simulink model "power_measure"  (Simulink 8.1)
settings: Solver=ode45  StartTime=0.0  StopTime=0.5  RelTol=1e-3
values from neighbouring files (symbols this model uses):
  sample = 10e-5    (= 0.0001)    [Symmetry_ini_COPY.m]    (also in animated_norms.m)
libraries: commsequence2 x12, powerlib x8, dspxfrm3 x6, aerolibconvert2 x2
settings Model: Creator=Neukirchner László  LastModifiedBy=Neukirchner László
settings DataIOCC: SignalLoggingSaveFormat=Dataset
settings OptimizationCC: ExpressionDepthLimit=128
settings DebuggingCC: FcnCallInpInsideContextMsg=EnableAllAsError
settings GRTTargetCC: CombineOutputUpdateFcns=on  GRTInterface=off

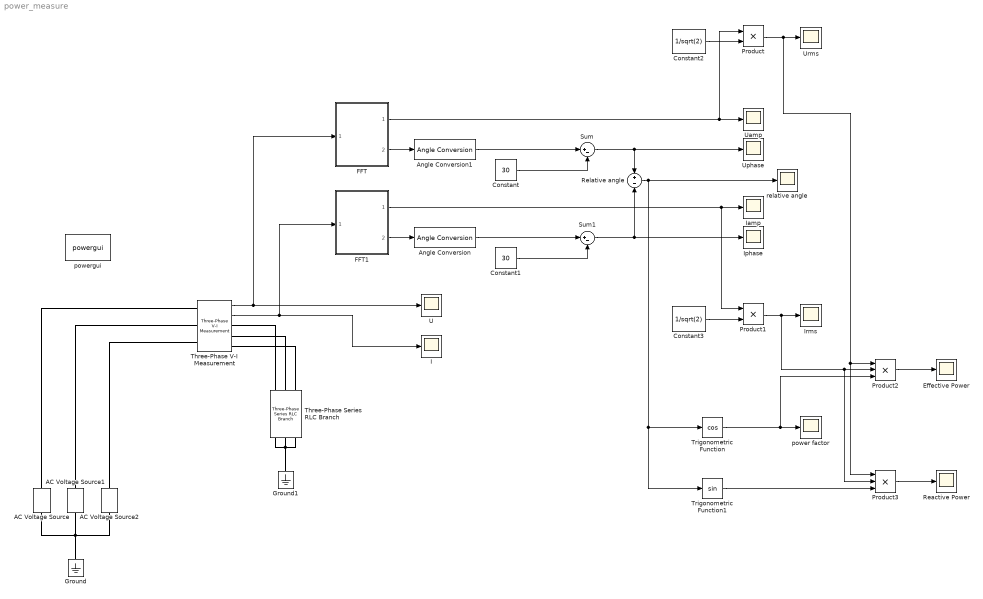
== system power_measure ==
  AC Voltage Source : powerlib/Electrical Sources/AC Voltage Source  Amplitude=325  Phase=0  Frequency=50  SampleTime=0  Measurements=None
  AC Voltage Source1 : powerlib/Electrical Sources/AC Voltage Source  Amplitude=325  Phase=-120  Frequency=50  SampleTime=0  Measurements=None
  AC Voltage Source2 : powerlib/Electrical Sources/AC Voltage Source  Amplitude=325  Phase=-240  Frequency=50  SampleTime=0  Measurements=None
  Angle Conversion : aerolibconvert2/Angle Conversion  IU=rad  OU=deg
  Angle Conversion1 : aerolibconvert2/Angle Conversion  IU=rad  OU=deg
  Constant : Constant  Value=30
  Constant1 : Constant  Value=30
  Constant2 : Constant  Value=1/sqrt(2)
  Constant3 : Constant  Value=1/sqrt(2)
  Effective Power : Scope
      settings: SaveName=ScopeData10
  FFT : Subsystem
  FFT1 : Subsystem
  Ground : powerlib/Elements/Ground  LConnTagsString=a
  Ground1 : powerlib/Elements/Ground  LConnTagsString=a
  I : Scope
  Iamp : Scope
      settings: SaveName=ScopeData4
  Iphase : Scope
      settings: SaveName=ScopeData5
  Irms : Scope
      settings: SaveName=ScopeData9
  Product : Product
  Product1 : Product
  Product2 : Product  Inputs=3
  Product3 : Product  Inputs=3
  Reactive Power : Scope
      settings: SaveName=ScopeData11
  Relative angle : Sum  Inputs=+|-
  Sum : Sum  Inputs=|+-
  Sum1 : Sum  Inputs=|+-
  Three-Phase Series RLC Branch : powerlib/Elements/Three-Phase Series RLC Branch  LConnTagsString=A|B|C  RConnTagsString=A|B|C  BranchType=RL  Resistance=100  Inductance=1e-1  Capacitance=1e-3  Measurements=None
  Three-Phase V-I Measurement : powerlib/Measurements/Three-Phase V-I Measurement  VoltageMeasurement=phase-to-ground  SetLabelV=off  LabelV=Vabc  Vpu=off  VpuLL=off  CurrentMeasurement=yes  SetLabelI=off  LabelI=Iabc  Ipu=off  Pbase=100e6  Vbase=500e3  OutputType=Complex  PhasorSimulation=off  PSBequivalent=0
  Trigonometric Function : Trigonometry  Operator=cos
  Trigonometric Function1 : Trigonometry
  U : Scope
  Uamp : Scope
      settings: SaveName=ScopeData2
  Uphase : Scope
      settings: SaveName=ScopeData3
  Urms : Scope
      settings: SaveName=ScopeData8
  power factor : Scope
      settings: SaveName=ScopeData7
  powergui : powerlib/powergui  Priority=1  SimulationMode=Continuous  SolverType=Tustin  SampleTime=50e-6  frequency=60  SPID=off  DisableSnubberDevices=off  DisableRonSwitches=off  DisableVfSwitches=off  SwTol=0  Interpol=off  DisplayEquations=off  frequencyindice=50  Pbase=100e6  ErrMax=1e-4  Iterations=50  UnitsV=kV  UnitsW=MW  FunctionMessages=off  echomessages=off  HookPort=off  EnableUseOfTLC=off  x0status=blocks  RestoreLinks=warning  ResistiveCurrentMeasurement=off  Frange=[0:2:500]  Ylog=off  Xlog=on  ShowGrid=off  save=off  variable=ZData  ZoomFFT=off  StartTime=0.0  cycles=1  DisplayStyle=1  fundamental=60  FreqAxis=off  MaxFrequency=1000  frequencyindicesteady=1  RmsSteady=1  display=off  Ts=0  methode=off
  relative angle : Scope
      settings: SaveName=ScopeData6
  wires:
  Three-Phase V-I Measurement/1 -> FFT/1(Voltage_3Phase), U/1
  Three-Phase V-I Measurement/2 -> FFT1/1(Current_3Phase), I/1
  FFT/1(Amplitude) -> Product/1, Uamp/1
  FFT/2(Phase_in_rad) -> Angle Conversion1/1
  FFT1/1(Amplitude) -> Product1/1, Iamp/1
  FFT1/2(Phase_in_rad) -> Angle Conversion/1
  Constant/1 -> Sum/2
  Angle Conversion1/1 -> Sum/1
  Sum/1 -> Relative angle/1, Uphase/1
  Constant1/1 -> Sum1/2
  Angle Conversion/1 -> Sum1/1
  Sum1/1 -> Relative angle/2, Iphase/1
  Relative angle/1 -> relative angle/1, Trigonometric Function1/1, Trigonometric Function/1
  Trigonometric Function/1 -> Product2/3, power factor/1
  Constant2/1 -> Product/2
  Constant3/1 -> Product1/2
  Product/1 -> Product3/1, Product2/1, Urms/1
  Product1/1 -> Product3/2, Product2/2, Irms/1
  Product2/1 -> Effective Power/1
  Product3/1 -> Reactive Power/1
  Trigonometric Function1/1 -> Product3/3
  connections:
  AC Voltage Source/LConn1 -- AC Voltage Source1/LConn1 -- AC Voltage Source2/LConn1 -- Ground/LConn1
  Three-Phase Series RLC Branch/RConn1 -- Ground1/LConn1 -- Three-Phase Series RLC Branch/RConn2 -- Three-Phase Series RLC Branch/RConn3
  Three-Phase V-I Measurement/RConn1 -- Three-Phase Series RLC Branch/LConn1
  Three-Phase V-I Measurement/RConn2 -- Three-Phase Series RLC Branch/LConn2
  Three-Phase V-I Measurement/RConn3 -- Three-Phase Series RLC Branch/LConn3
  AC Voltage Source/RConn1 -- Three-Phase V-I Measurement/LConn1
  AC Voltage Source1/RConn1 -- Three-Phase V-I Measurement/LConn2
  AC Voltage Source2/RConn1 -- Three-Phase V-I Measurement/LConn3

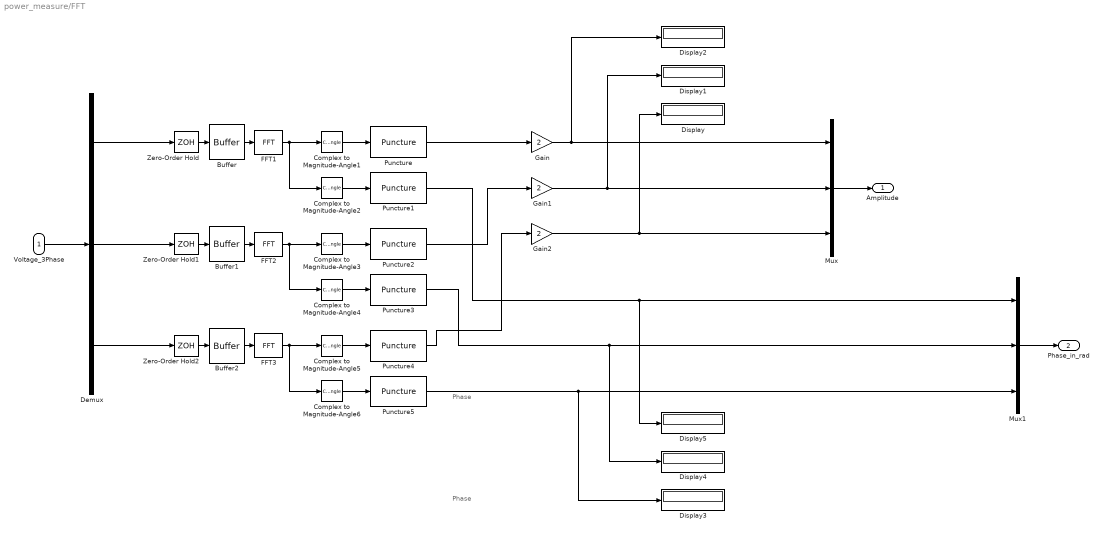
== system power_measure/FFT ==
  note: Phase
  note: Phase
  Voltage_3Phase : Inport
  Buffer : Buffer  N=128  TreatMby1Signals=One channel
  Buffer1 : Buffer  N=128  TreatMby1Signals=One channel
  Buffer2 : Buffer  N=128  TreatMby1Signals=One channel
  Complex to Magnitude-Angle1 : ComplexToMagnitudeAngle  Output=Magnitude
  Complex to Magnitude-Angle2 : ComplexToMagnitudeAngle  Output=Angle
  Complex to Magnitude-Angle3 : ComplexToMagnitudeAngle  Output=Magnitude
  Complex to Magnitude-Angle4 : ComplexToMagnitudeAngle  Output=Angle
  Complex to Magnitude-Angle5 : ComplexToMagnitudeAngle  Output=Magnitude
  Complex to Magnitude-Angle6 : ComplexToMagnitudeAngle  Output=Angle
  Demux : Demux  Outputs=3
  Display{,1..5} (6 alike) : Display
  FFT1 : dspxfrm3/FFT  CompMethod=Table lookup  TableOpt=NEW  TableOptActive=Speed  BitRevOrder=off  InheritFFTLength=on  FFTLength=64  RowConvenienceOn=on  FFTImplementation=Auto  SkipNorm=on  firstCoeffDataTypeStr=Inherit: Same word length as input  firstCoeffLastDataTypeStr=Inherit: Same word length as input  outputMin=[]  outputMax=[]  roundingMode=Floor  overflowMode=off
  FFT2 : dspxfrm3/FFT  CompMethod=Table lookup  TableOpt=NEW  TableOptActive=Speed  BitRevOrder=off  InheritFFTLength=on  FFTLength=64  RowConvenienceOn=on  FFTImplementation=Auto  SkipNorm=on  firstCoeffDataTypeStr=Inherit: Same word length as input  firstCoeffLastDataTypeStr=Inherit: Same word length as input  outputMin=[]  outputMax=[]  roundingMode=Floor  overflowMode=off
  FFT3 : dspxfrm3/FFT  CompMethod=Table lookup  TableOpt=NEW  TableOptActive=Speed  BitRevOrder=off  InheritFFTLength=on  FFTLength=64  RowConvenienceOn=on  FFTImplementation=Auto  SkipNorm=on  firstCoeffDataTypeStr=Inherit: Same word length as input  firstCoeffLastDataTypeStr=Inherit: Same word length as input  outputMin=[]  outputMax=[]  roundingMode=Floor  overflowMode=off
  Gain : Gain  Gain=2  SampleTime=sample
  Gain1 : Gain  Gain=2  SampleTime=sample
  Gain2 : Gain  Gain=2  SampleTime=sample
  Mux : Mux  Inputs=3
  Mux1 : Mux  Inputs=3
  Puncture{,1..5} (6 alike) : commsequence2/Puncture  punctureVector=s'
  Zero-Order Hold : ZeroOrderHold  SampleTime=20e-3/128
  Zero-Order Hold1 : ZeroOrderHold  SampleTime=20e-3/128
  Zero-Order Hold2 : ZeroOrderHold  SampleTime=20e-3/128
  Amplitude : Outport
  Phase_in_rad : Outport  Port=2
  wires:
  FFT1/1 -> Complex to Magnitude-Angle1/1, Complex to Magnitude-Angle2/1
  Buffer/1 -> FFT1/1
  Zero-Order Hold/1 -> Buffer/1
  Complex to Magnitude-Angle1/1 -> Puncture/1
  Complex to Magnitude-Angle2/1 -> Puncture1/1
  FFT2/1 -> Complex to Magnitude-Angle4/1, Complex to Magnitude-Angle3/1
  Buffer1/1 -> FFT2/1
  Zero-Order Hold1/1 -> Buffer1/1
  Complex to Magnitude-Angle3/1 -> Puncture2/1
  Complex to Magnitude-Angle4/1 -> Puncture3/1
  FFT3/1 -> Complex to Magnitude-Angle5/1, Complex to Magnitude-Angle6/1
  Buffer2/1 -> FFT3/1
  Zero-Order Hold2/1 -> Buffer2/1
  Complex to Magnitude-Angle5/1 -> Puncture4/1
  Complex to Magnitude-Angle6/1 -> Puncture5/1
  Voltage_3Phase/1 -> Demux/1
  Demux/2 -> Zero-Order Hold1/1
  Demux/3 -> Zero-Order Hold2/1
  Puncture/1 -> Gain/1
  Puncture2/1 -> Gain1/1
  Puncture4/1 -> Gain2/1
  Puncture1/1 -> Display5/1, Mux1/1
  Puncture3/1 -> Display4/1, Mux1/2
  Puncture5/1 -> Display3/1, Mux1/3
  Mux/1 -> Amplitude/1
  Mux1/1 -> Phase_in_rad/1
  Gain/1 -> Display2/1, Mux/1
  Gain1/1 -> Display1/1, Mux/2
  Gain2/1 -> Display/1, Mux/3
  Demux/1 -> Zero-Order Hold/1

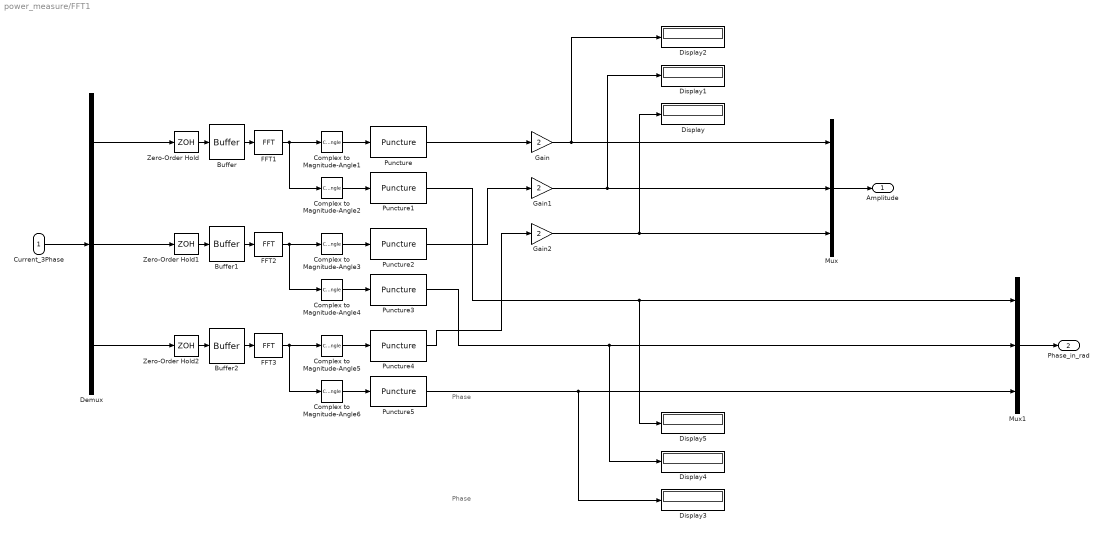
== system power_measure/FFT1 ==
  note: Phase
  note: Phase
  Current_3Phase : Inport
  Buffer : Buffer  N=128  TreatMby1Signals=One channel
  Buffer1 : Buffer  N=128  TreatMby1Signals=One channel
  Buffer2 : Buffer  N=128  TreatMby1Signals=One channel
  Complex to Magnitude-Angle1 : ComplexToMagnitudeAngle  Output=Magnitude
  Complex to Magnitude-Angle2 : ComplexToMagnitudeAngle  Output=Angle
  Complex to Magnitude-Angle3 : ComplexToMagnitudeAngle  Output=Magnitude
  Complex to Magnitude-Angle4 : ComplexToMagnitudeAngle  Output=Angle
  Complex to Magnitude-Angle5 : ComplexToMagnitudeAngle  Output=Magnitude
  Complex to Magnitude-Angle6 : ComplexToMagnitudeAngle  Output=Angle
  Demux : Demux  Outputs=3
  Display{,1..5} (6 alike) : Display
  FFT1 : dspxfrm3/FFT  CompMethod=Table lookup  TableOpt=NEW  TableOptActive=Speed  BitRevOrder=off  InheritFFTLength=on  FFTLength=64  RowConvenienceOn=on  FFTImplementation=Auto  SkipNorm=on  firstCoeffDataTypeStr=Inherit: Same word length as input  firstCoeffLastDataTypeStr=Inherit: Same word length as input  outputMin=[]  outputMax=[]  roundingMode=Floor  overflowMode=off
  FFT2 : dspxfrm3/FFT  CompMethod=Table lookup  TableOpt=NEW  TableOptActive=Speed  BitRevOrder=off  InheritFFTLength=on  FFTLength=64  RowConvenienceOn=on  FFTImplementation=Auto  SkipNorm=on  firstCoeffDataTypeStr=Inherit: Same word length as input  firstCoeffLastDataTypeStr=Inherit: Same word length as input  outputMin=[]  outputMax=[]  roundingMode=Floor  overflowMode=off
  FFT3 : dspxfrm3/FFT  CompMethod=Table lookup  TableOpt=NEW  TableOptActive=Speed  BitRevOrder=off  InheritFFTLength=on  FFTLength=64  RowConvenienceOn=on  FFTImplementation=Auto  SkipNorm=on  firstCoeffDataTypeStr=Inherit: Same word length as input  firstCoeffLastDataTypeStr=Inherit: Same word length as input  outputMin=[]  outputMax=[]  roundingMode=Floor  overflowMode=off
  Gain : Gain  Gain=2  SampleTime=sample
  Gain1 : Gain  Gain=2  SampleTime=sample
  Gain2 : Gain  Gain=2  SampleTime=sample
  Mux : Mux  Inputs=3
  Mux1 : Mux  Inputs=3
  Puncture{,1..5} (6 alike) : commsequence2/Puncture  punctureVector=s'
  Zero-Order Hold : ZeroOrderHold  SampleTime=20e-3/128
  Zero-Order Hold1 : ZeroOrderHold  SampleTime=20e-3/128
  Zero-Order Hold2 : ZeroOrderHold  SampleTime=20e-3/128
  Amplitude : Outport
  Phase_in_rad : Outport  Port=2
  wires:
  Demux/1 -> Zero-Order Hold/1
  Gain2/1 -> Mux/3, Display/1
  Gain1/1 -> Mux/2, Display1/1
  Gain/1 -> Mux/1, Display2/1
  Mux1/1 -> Phase_in_rad/1
  Mux/1 -> Amplitude/1
  Puncture5/1 -> Mux1/3, Display3/1
  Puncture3/1 -> Mux1/2, Display4/1
  Puncture1/1 -> Mux1/1, Display5/1
  Puncture4/1 -> Gain2/1
  Puncture2/1 -> Gain1/1
  Puncture/1 -> Gain/1
  Demux/3 -> Zero-Order Hold2/1
  Demux/2 -> Zero-Order Hold1/1
  Current_3Phase/1 -> Demux/1
  Complex to Magnitude-Angle6/1 -> Puncture5/1
  Complex to Magnitude-Angle5/1 -> Puncture4/1
  Zero-Order Hold2/1 -> Buffer2/1
  Buffer2/1 -> FFT3/1
  FFT3/1 -> Complex to Magnitude-Angle6/1, Complex to Magnitude-Angle5/1
  Complex to Magnitude-Angle4/1 -> Puncture3/1
  Complex to Magnitude-Angle3/1 -> Puncture2/1
  Zero-Order Hold1/1 -> Buffer1/1
  Buffer1/1 -> FFT2/1
  FFT2/1 -> Complex to Magnitude-Angle3/1, Complex to Magnitude-Angle4/1
  Complex to Magnitude-Angle2/1 -> Puncture1/1
  Complex to Magnitude-Angle1/1 -> Puncture/1
  Zero-Order Hold/1 -> Buffer/1
  Buffer/1 -> FFT1/1
  FFT1/1 -> Complex to Magnitude-Angle2/1, Complex to Magnitude-Angle1/1
